simulink model "Transformer_Diff_Relay"  (R2024b)
settings: Solver=ode45  StartTime=0.0  StopTime=0.3  RelTol=1e-3  EnableMultiTasking=on
libraries: spsThreePhaseVIMeasurementLib x2, spsThreePhaseBreakerLib x2, spsThreePhaseFaultLib x2, spsThreePhaseSeriesRLCLoadLib x1, spsThreePhaseTransformerTwoWindingsLib x1, spsThreePhaseSourceLib x1, spspowerguiLib x1
settings Model: Creator=e508034  LastModifiedBy=Aaahm
settings SolverCC: AlgebraicLoopSolver=TrustRegion
settings DataIOCC: LimitDataPoints=on  SaveFormat=Array  SignalLoggingSaveFormat=ModelDataLogs  ReturnWorkspaceOutputs=off
settings OptimizationCC: ExpressionDepthLimit=2147483647  LifeSpan=inf
settings DebuggingCC: AlgebraicLoopMsg=none  UnderspecifiedInitializationDetection=Classic  MergeDetectMultiDrivingBlocksExec=none  SolverPrmCheckMsg=warning  FcnCallInpInsideContextMsg=warning  UnconnectedInputMsg=warning  UnconnectedOutputMsg=warning  UnconnectedLineMsg=warning  StateNameClashWarn=warning  SFUnexpectedBacktrackingDiag=warning  SFNoUnconditionalDefaultTransitionDiag=warning  SFExecutionAtInitializationDiag=none  ArithmeticOperatorsInVariantConditions=warning
settings HardwareCC: ProdBitPerPointer=32  ProdBitPerSizeT=32  ProdBitPerPtrDiffT=32  ProdLargestAtomicFloat=None  ProdIntDivRoundTo=Undefined  ProdEndianess=Unspecified  ProdWordSize=32  ProdHWDeviceType=32-bit Generic
settings ModelReferenceCC: PropagateSignalLabelsOutOfModel=off
settings SFSimCC: SimUseLocalCustomCode=off  CustomCodeUndefinedFunction=UseInterfaceOnly
settings RTWCC: RTWUseLocalCustomCode=off  GPUComputeCapability=3.5
settings CodeAppCC: StateflowObjectComments=on
settings GRTTargetCC: TargetLangStandard=C89/C90 (ANSI)  CombineOutputUpdateFcns=off  GRTInterface=on
settings ConfigComp: CovMetricSettings=dw  CovSaveCumulativeToWorkspaceVar=on  CovSaveSingleToWorkspaceVar=on  CovExternalEMLEnable=off

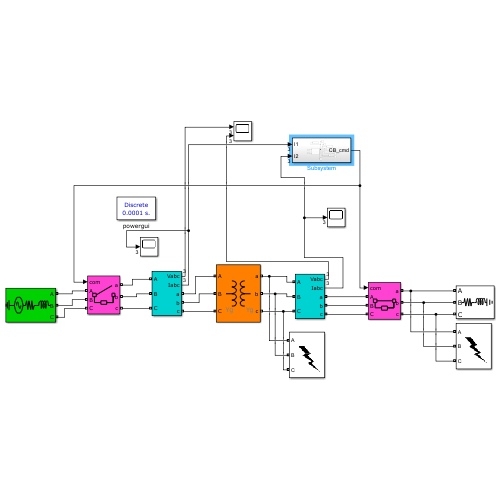
[thumbnail: Simulink's stored preview of the top-level diagram]
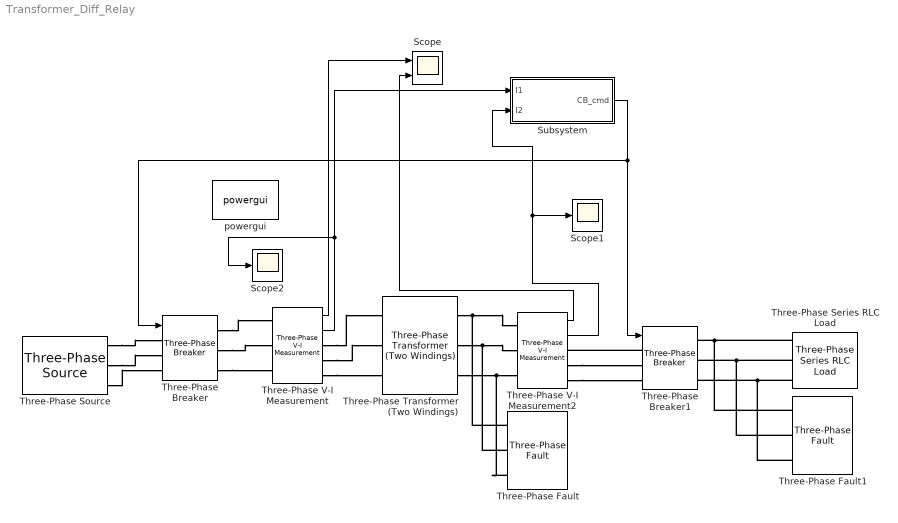
== system Transformer_Diff_Relay ==
  Scope : Scope  NumInputPorts=2
  Scope1 : Scope
  Scope2 : Scope
  Subsystem : Subsystem
  Three-Phase Series RLC Load : spsThreePhaseSeriesRLCLoadLib/Three-Phase Series RLC Load  LConnTagsString=A|B|C  Configuration=Y (grounded)  NominalVoltage=33e3  Vabc=[1e3 1e3 1e3]  Vabcp=[1e3 1e3 1e3]  NominalFrequency=50  UnbalancedPower=off  ActivePower=150e3  InductivePower=50e3  CapacitivePower=0  Pabc=[10e3 9e3 11e3]  QLabc=[100 90 110]  QCabc=[100 90 110]  Pabcp=[10e3 9e3 11e3]  QLabcp=[100 90 110]  QCabcp=[100 90 110]  Measurements=None  LoadType=constant Z
  Three-Phase Transformer (Two Windings) : spsThreePhaseTransformerTwoWindingsLib/Three-Phase Transformer (Two Windings)  Winding1Connection=Yg  Winding2Connection=Yg  CoreType=Three single-phase transformers  SetSaturation=off  Hysteresis=off  DataFile='hysteresis'  SetInitialFlux=off  Measurements=None  UNITS=pu  NominalPower=[ 200e6 , 50 ]  Winding1=[ 11e3 , 0.002 , 0.8 ]  Winding2=[ 33e3 , 0.002 , 0.8 ]  Rm=200  Lm=200  L0=0.5  Saturation=[ 0,0 ; 0.0024,1.2 ; 1.0,1.52 ]  InitialFluxes=[-0.000104815018313083 4.84621187988385e-05 5.63528995142447e-05]  BreakLoop=off  DiscreteSolver=Trapezoidal iterative  DataType=off  TransfoNumber=1
  Three-Phase V-I Measurement : spsThreePhaseVIMeasurementLib/Three-Phase V-I Measurement  VoltageMeasurement=phase-to-ground  SetLabelV=off  LabelV=Vabc  Vpu=off  VpuLL=off  CurrentMeasurement=yes  SetLabelI=off  LabelI=Iabc  Ipu=on  Pbase=200e6  Vbase=11e3  OutputType=Complex  PhasorSimulation=off  PSBequivalent=0
  Three-Phase V-I Measurement2 : spsThreePhaseVIMeasurementLib/Three-Phase V-I Measurement  VoltageMeasurement=phase-to-ground  SetLabelV=off  LabelV=Vabc  Vpu=off  VpuLL=off  CurrentMeasurement=yes  SetLabelI=off  LabelI=Iabc  Ipu=on  Pbase=200e6  Vbase=33e3  OutputType=Complex  PhasorSimulation=off  PSBequivalent=0
  Three-Phase Breaker : spsThreePhaseBreakerLib/Three-Phase Breaker  InitialState=open  SwitchA=on  SwitchB=on  SwitchC=on  SwitchTimes=[0.1]  External=on  BreakerResistance=0.001  SnubberResistance=1e6  SnubberCapacitance=inf  Measurements=None
  Three-Phase Breaker1 : spsThreePhaseBreakerLib/Three-Phase Breaker  InitialState=closed  SwitchA=on  SwitchB=on  SwitchC=on  SwitchTimes="[4/60  10/60]"  External=on  BreakerResistance=0.001  SnubberResistance=1e6  SnubberCapacitance=inf  Measurements=None
  Three-Phase Fault : spsThreePhaseFaultLib/Three-Phase Fault  InitialStates=0  FaultA=on  FaultB=on  FaultC=on  GroundFault=on  SwitchTimes=[0.1]  External=off  SwitchStatus=NaN  FaultResistance=0.001  GroundResistance=0.01  SnubberResistance=1e6  SnubberCapacitance=inf  Measurements=None
  Three-Phase Fault1 : spsThreePhaseFaultLib/Three-Phase Fault  InitialStates=0  FaultA=off  FaultB=off  FaultC=off  GroundFault=off  SwitchTimes=[0.2]  External=off  SwitchStatus=NaN  FaultResistance=0.001  GroundResistance=0.01  SnubberResistance=1e6  SnubberCapacitance=inf  Measurements=None
  Three-Phase Source : spsThreePhaseSourceLib/Three-Phase Source  InternalConnection=Yg  VoltagePhases=off  Voltage=11e3  PhaseAngle=0  Voltage_phases=[25e3 25e3 25e3]/sqrt(3)  PhaseAngles_phases=[0 -120 +120]  Frequency=50  NonIdealSource=on  SpecifyImpedance=on  Resistance=0.8929  Inductance=16.58e-3  ShortCircuitLevel=500e6  BaseVoltage=11e3  XRratio=7  BusType=swing  Pref=10e3  Qref=0  Prefabc=[10e3, 10e3, 10e3]  Qrefabc=[0, 0, 0]  Qmin=-inf  Qmax=inf
  powergui : spspowerguiLib/powergui  Priority=1  SimulationMode=Discrete  SampleTime=1e-4  frequency=60  Iterations=50  frequencyindice=50  Pbase=100e6  ErrMax=1e-4  UnitsV=kV  UnitsW=MW  buscounter=0  FunctionMessages=off  echomessages=off  EnableUseOfTLC=off  CurrentSourceSwitches=off  DisableSnubberDevices=off  DisableRonSwitches=off  DisableVfSwitches=off  DisplayEquations=off  AutomaticDiscreteSolvers=off  SolverType=Tustin/Backward Euler (TBE)  Interpol=off  ExternalGateDelay=off  methode=off  Ts=0  x0status=blocks  SPID=off  SwTol=0  HookPort=off  NonlinearTolerance=1e-4  nMaxIteration=100  ContinueOnMaxIteration=off  RestoreLinks=warning  ResistiveCurrentMeasurement=off  Frange=[0:2:500]  Ylog=off  Xlog=on  ShowGrid=off  save=off  variable=ZData  structure=0  ZoomFFT=on  StartTime=0.0  cycles=1  DisplayStyle=1  fundamental=60  FreqAxis=off  MaxFrequency=1000  frequencyindicesteady=1  RmsSteady=1  display=off
  wires:
  Three-Phase V-I Measurement/1 -> Scope/1
  Three-Phase V-I Measurement/2 -> Scope2/1, Subsystem/1(I1)
  Three-Phase V-I Measurement2/1 -> Scope/2
  Three-Phase V-I Measurement2/2 -> Scope1/1, Subsystem/2(I2)
  Subsystem/1(CB_cmd) -> Three-Phase Breaker/1, Three-Phase Breaker1/1
  connections:
  Three-Phase Breaker/RConn1 -- Three-Phase V-I Measurement/LConn1
  Three-Phase Breaker/RConn2 -- Three-Phase V-I Measurement/LConn2
  Three-Phase Breaker/RConn3 -- Three-Phase V-I Measurement/LConn3
  Three-Phase V-I Measurement/RConn1 -- Three-Phase Transformer (Two Windings)/LConn1
  Three-Phase V-I Measurement/RConn2 -- Three-Phase Transformer (Two Windings)/LConn2
  Three-Phase V-I Measurement/RConn3 -- Three-Phase Transformer (Two Windings)/LConn3
  Three-Phase Transformer (Two Windings)/RConn1 -- Three-Phase Fault/LConn1 -- Three-Phase V-I Measurement2/LConn1
  Three-Phase Transformer (Two Windings)/RConn2 -- Three-Phase Fault/LConn2 -- Three-Phase V-I Measurement2/LConn2
  Three-Phase Transformer (Two Windings)/RConn3 -- Three-Phase Fault/LConn3 -- Three-Phase V-I Measurement2/LConn3
  Three-Phase Breaker1/LConn1 -- Three-Phase V-I Measurement2/RConn1
  Three-Phase V-I Measurement2/RConn3 -- Three-Phase Breaker1/LConn3
  Three-Phase V-I Measurement2/RConn2 -- Three-Phase Breaker1/LConn2
  Three-Phase Series RLC Load/LConn1 -- Three-Phase Fault1/LConn1 -- Three-Phase Breaker1/RConn1
  Three-Phase Series RLC Load/LConn2 -- Three-Phase Fault1/LConn2 -- Three-Phase Breaker1/RConn2
  Three-Phase Series RLC Load/LConn3 -- Three-Phase Fault1/LConn3 -- Three-Phase Breaker1/RConn3
  Three-Phase Source/RConn1 -- Three-Phase Breaker/LConn1
  Three-Phase Source/RConn2 -- Three-Phase Breaker/LConn2
  Three-Phase Source/RConn3 -- Three-Phase Breaker/LConn3

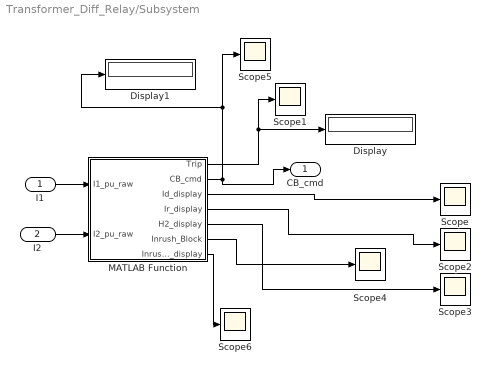
== system Transformer_Diff_Relay/Subsystem ==
  I1 : Inport
  I2 : Inport  Port=2
  Display : Display
  Display1 : Display
  MATLAB Function : MATLAB Function  TreatAsAtomicUnit=on
  Scope{,1..6} (7 alike) : Scope
  CB_cmd : Outport
  wires:
  MATLAB Function/3(Id_display) -> Scope/1
  MATLAB Function/1(Trip) -> Scope1/1, Display/1
  I1/1 -> MATLAB Function/1(I1_pu_raw)
  I2/1 -> MATLAB Function/2(I2_pu_raw)
  MATLAB Function/4(Ir_display) -> Scope2/1
  MATLAB Function/5(H2_display) -> Scope3/1
  MATLAB Function/6(Inrush_Block) -> Scope4/1
  MATLAB Function/2(CB_cmd) -> CB_cmd/1, Display1/1, Scope5/1
  MATLAB Function/7(Inrush_Current_display) -> Scope6/1

== matlab function Transformer_Diff_Relay/Subsystem/MATLAB Function ==
  data: I1_pu_raw input; Trip output; CB_cmd output; I2_pu_raw input; Id_display output; Ir_display output; H2_display output; Inrush_Block output; Inrush_Current_display output
function [Trip, CB_cmd, Id_display, Ir_display, H2_display, Inrush_Block, Inrush_Current_display] = Relay_advanced(I1_pu_raw, I2_pu_raw)
persistent buf1 buf2 k trip_latch polarity_ready pol trip_counter

%% Simulation parameters
Ts = 1e-4;                 % powergui sample time
f0 = 50;                   % system frequency
N  = round(1/(f0*Ts));     % samples per cycle = 200

%% Relay settings
startup_block_time = 0.08;
startup_samples    = round(startup_block_time/Ts);

Id_pickup = 0.25;          % pu minimum pickup
Slope1    = 0.30;
Slope2    = 0.70;
Ir_break  = 1.50;          % pu

HighSet = 6.00;            % pu instantaneous differential trip

H2_block_ratio = 0.15;     % second harmonic inrush blocking
H5_block_ratio = 0.25;     % fifth harmonic overexcitation blocking

confirm_time    = 0.005;   % 5 ms confirmation time
confirm_samples = round(confirm_time/Ts);

%% Initialize
if isempty(buf1)
    buf1 = zeros(N,3);
    buf2 = zeros(N,3);
    k = 0;
    trip_latch = 0;
    polarity_ready = 0;
    pol = 1;
    trip_counter = 0;
end

%% Default outputs
Trip = trip_latch;
CB_cmd = 1 - Trip;

Id_display = 0;
Ir_display = 0;
H2_display = 0;
Inrush_Block = 0;
Inrush_Current_display = 0;

%% Input formatting
I1 = reshape(I1_pu_raw, 1, []);
I2 = reshape(I2_pu_raw, 1, []);

if length(I1) < 3 || length(I2) < 3
    Trip = 0;
    CB_cmd = 1;
    Id_display = 0;
    Ir_display = 0;
    H2_display = 0;
    Inrush_Block = 0;
    Inrush_Current_display = 0;
    return;
end

I1 = I1(1:3);
I2 = I2(1:3);

%% Inrush current display signal
% This output shows the instantaneous primary-side current magnitude.
% It is useful for observing the current behavior during transformer energization.
Inrush_Current_display = max(abs(I1));

%% Buffer update
k = k + 1;
idx = mod(k-1, N) + 1;

buf1(idx,:) = I1;
buf2(idx,:) = I2;

%% Wait until one full cycle is available
if k < N
    Trip = trip_latch;
    CB_cmd = 1 - Trip;
    Id_display = 0;
    Ir_display = 0;
    H2_display = 0;
    Inrush_Block = 0;
    return;
end

%% Arrange one-cycle window
if idx == N
    x1 = buf1;
    x2 = buf2;
else
    x1 = [buf1(idx+1:end,:); buf1(1:idx,:)];
    x2 = [buf2(idx+1:end,:); buf2(1:idx,:)];
end

%% DFT phasors
I1_1 = local_dft(x1, 1, N);   % fundamental
I2_1 = local_dft(x2, 1, N);

I1_2 = local_dft(x1, 2, N);   % second harmonic
I2_2 = local_dft(x2, 2, N);

I1_5 = local_dft(x1, 5, N);   % fifth harmonic
I2_5 = local_dft(x2, 5, N);

%% Automatic polarity correction
% This selects the correct secondary current direction during the initial healthy period.
if polarity_ready == 0 && k > N && k < startup_samples

    error_same_direction     = sum(abs(I1_1 - I2_1));
    error_opposite_direction = sum(abs(I1_1 + I2_1));

    if error_same_direction <= error_opposite_direction
        pol = 1;
    else
        pol = -1;
    end

    polarity_ready = 1;
end

I2c_1 = pol * I2_1;
I2c_2 = pol * I2_2;
I2c_5 = pol * I2_5;

%% Differential and restraint currents
Id_phase = abs(I1_1 - I2c_1);
Ir_phase = 0.5 * (abs(I1_1) + abs(I2c_1));

Id_display = max(Id_phase);
Ir_display = max(Ir_phase);

%% Harmonic ratios
Id2_phase = abs(I1_2 - I2c_2);
Id5_phase = abs(I1_5 - I2c_5);

H2_ratio = zeros(1,3);
H5_ratio = zeros(1,3);

for ph = 1:3
    if Id_phase(ph) > 1e-6
        H2_ratio(ph) = Id2_phase(ph) / Id_phase(ph);
        H5_ratio(ph) = Id5_phase(ph) / Id_phase(ph);
    else
        H2_ratio(ph) = 0;
        H5_ratio(ph) = 0;
    end
end

H2_display = max(H2_ratio);

if H2_display > H2_block_ratio
    Inrush_Block = 1;
else
    Inrush_Block = 0;
end

%% Differential operation logic
Diff_Operate = 0;
HighSet_Trip = 0;

for ph = 1:3

    Id = Id_phase(ph);
    Ir = Ir_phase(ph);

    if Ir <= Ir_break
        threshold = Id_pickup + Slope1 * Ir;
    else
        threshold = Id_pickup + Slope1 * Ir_break + Slope2 * (Ir - Ir_break);
    end

    phase_inrush_block = H2_ratio(ph) > H2_block_ratio;
    phase_overexc_block = H5_ratio(ph) > H5_block_ratio;

    normal_diff_condition = (Id > threshold) && ~phase_inrush_block && ~phase_overexc_block;
    highset_condition = Id > HighSet;

    if normal_diff_condition
        Diff_Operate = 1;
    end

    if highset_condition
        HighSet_Trip = 1;
    end
end

%% Startup blocking
if k < startup_samples
    Diff_Operate = 0;
    HighSet_Trip = 0;
    Inrush_Block = 0;
end

%% Final trip with confirmation time
operate = Diff_Operate || HighSet_Trip;

if operate == 1
    trip_counter = trip_counter + 1;
else
    trip_counter = 0;
end

if trip_counter >= confirm_samples
    trip_latch = 1;
end

Trip = trip_latch;

% Breaker command:
% 1 = Closed
% 0 = Open
CB_cmd = 1 - Trip;

end

%% ==========================================================
function phasor = local_dft(x, h, N)
% RMS complex phasor for harmonic order h
% x size: N x 3

phasor = complex(zeros(1,3), zeros(1,3));

n = 0:N-1;
w = exp(-1i * 2*pi*h*n/N).';

for ph = 1:3
    temp = (sqrt(2)/N) * sum(x(:,ph) .* w);
    phasor(ph) = complex(temp);
end

end
